simulink model "VDSE_2018a"  (R2018a)
settings: Solver=ode5  StartTime=0.0  StopTime=T_simulation  FixedStep=simulation_step_time  RelTol=1e-3
values from neighbouring files (symbols this model uses):
  A = 2    [vehicle_parameters_script.m]
  bump_height = 0    [vehicle_parameters_script.m]
  bump_length = 1    [vehicle_parameters_script.m]
  bump_time = 1    [vehicle_parameters_script.m]
  Bxf = 17.156    [BCD_Parameters.m]
  Bxr = 17.156    [BCD_Parameters.m]
  Byf = 12.71    [BCD_Parameters.m]
  Byr = 12.71    [BCD_Parameters.m]
  cd = 0.35    [vehicle_parameters_script.m]
  central_diff = 1    [vehicle_parameters_script.m]
  cF = 5000    [vehicle_parameters_script.m]
  clF = -0.15    [vehicle_parameters_script.m]
  clR = -0.20    (= -0.2)    [vehicle_parameters_script.m]
  cp_FA = 30    [vehicle_parameters_script.m]
  cp_RA = 13    [vehicle_parameters_script.m]
  cR = 5000    [vehicle_parameters_script.m]
  ctF = tireF.VERTICAL_DAMPING    [vehicle_parameters_script.m]
  ctR = tireR.VERTICAL_DAMPING    [vehicle_parameters_script.m]
  Cxf = 1.406    [BCD_Parameters.m]
  Cxr = 1.406    [BCD_Parameters.m]
  Cyf = 1.63    [BCD_Parameters.m]
  Cyr = 1.63    [BCD_Parameters.m]
  Dxf = 1.2    [BCD_Parameters.m]
  Dxr = 1.2    [BCD_Parameters.m]
  Dyf = 1.1    [BCD_Parameters.m]
  Dyr = 1.8    [BCD_Parameters.m]
  enableDriverControl = 0    [vehicle_parameters_script.m]
  enableLongDynamics = 1    [vehicle_parameters_script.m]
  enablePowertrain = 1    [vehicle_parameters_script.m]
  front_dr = 3.8    [vehicle_parameters_script.m]
  g = 9.806    [vehicle_parameters_script.m]
  Gear_numbers = [1 2 3 4 5 6]    [vehicle_parameters_script.m]
  GR = [2.9 1.8 1.3 1 0.85 0.75]    [vehicle_parameters_script.m]
  hcog = 0.5    [vehicle_parameters_script.m]
  hpc = 0.0    (= 0)    [vehicle_parameters_script.m]
  hrcF = 0.3    [vehicle_parameters_script.m]
  hrcg = (hrcF*lR+hrcR*lF)/(lF+lR)    (= 0.25108)    [vehicle_parameters_script.m]
  hrcR = 0.2    [vehicle_parameters_script.m]
  huFcog = 0.32    [vehicle_parameters_script.m]
  huRcog = 0.32    [vehicle_parameters_script.m]
  initial_gear = 1    [vehicle_parameters_script.m]
  JwF = 2.45    [vehicle_parameters_script.m]
  JwR = 2.45    [vehicle_parameters_script.m]
  Jx = 430    [vehicle_parameters_script.m]
  Jy = 1309    [vehicle_parameters_script.m]
  Jz = 1461    [vehicle_parameters_script.m]
  kF = 40000    [vehicle_parameters_script.m]
  kR = 35000    [vehicle_parameters_script.m]
  kRF = 0    [vehicle_parameters_script.m]
  kRR = 0    [vehicle_parameters_script.m]
  ktF = tireF.VERTICAL_STIFFNESS    [vehicle_parameters_script.m]
  ktR = tireR.VERTICAL_STIFFNESS    [vehicle_parameters_script.m]
  lF = 1.223    [vehicle_parameters_script.m]
  lR = l-lF    (= 1.277)    [vehicle_parameters_script.m]
  m = 1310    [vehicle_parameters_script.m]
  max_pressure = 1000    [vehicle_parameters_script.m]
  maxrpm = 4000    [vehicle_parameters_script.m]
  mF = 45    [vehicle_parameters_script.m]
  minrpm = 1500    [vehicle_parameters_script.m]
  mR = 50    [vehicle_parameters_script.m]
  output_samping_time = 0.001    [vehicle_parameters_script.m]
  phi0 = 0    [vehicle_parameters_script.m]
  phi_dot0 = 0    [vehicle_parameters_script.m]
  psi0 = 0    [vehicle_parameters_script.m]
  psi_dot0 = 0    [vehicle_parameters_script.m]
  rear_dr = 3.8    [vehicle_parameters_script.m]
  requested_speed = 100/3.6    (= 27.7777777778)    [vehicle_parameters_script.m]
  rF = tireF.UNLOADED_RADIUS    [vehicle_parameters_script.m]
  rho = 1.2    [vehicle_parameters_script.m]
  RPMME = Engine(:,1)    [vehicle_parameters_script.m]
  rR = tireR.UNLOADED_RADIUS    [vehicle_parameters_script.m]
  steer_ratio = 13.25    [vehicle_parameters_script.m]
  TFL = 0    [vehicle_parameters_script.m]
  TFR = 0    [vehicle_parameters_script.m]
  theta0 = 0    [vehicle_parameters_script.m]
  theta_dot0 = 0    [vehicle_parameters_script.m]
  TorqueME = []    [vehicle_parameters_script.m]
  TRL = 0    [vehicle_parameters_script.m]
  TRR = 0    [vehicle_parameters_script.m]
  Vx0 = 100/3.6    (= 27.7777777778)    [vehicle_parameters_script.m]
  Vy0 = 0    [vehicle_parameters_script.m]
  Vz0 = 0    [vehicle_parameters_script.m]
  wF = 1.578    [vehicle_parameters_script.m]
  wR = 1.544    [vehicle_parameters_script.m]
  x0 = 0    [vehicle_parameters_script.m]
  xcog_overall = (2*mR*xR+2*xF*mF+m*xs)/(m+2*mF+2*mR)    (= 1.23475333333)    [vehicle_parameters_script.m]
  y0 = 0    [vehicle_parameters_script.m]
  z0 = 0    [vehicle_parameters_script.m]
  zFL0 = 0    [vehicle_parameters_script.m]
  zFL_dot0 = 0    [vehicle_parameters_script.m]
  zFR0 = 0    [vehicle_parameters_script.m]
  zFR_dot0 = 0    [vehicle_parameters_script.m]
  zRL0 = 0    [vehicle_parameters_script.m]
  zRL_dot0 = 0    [vehicle_parameters_script.m]
  zRR0 = 0    [vehicle_parameters_script.m]
  zRR_dot0 = 0    [vehicle_parameters_script.m]
undefined symbols (not defined in the file or in its folder): exf, exr, eyf, eyr, FNOMINf, FNOMINr, PCX1f, PCX1r, PCY1f, PCY1r, PDX1f, PDX1r, PDX2f, PDX2r, PDY1f, PDY1r, PDY2f, PDY2r, PDY3f, PDY3r, PEX1f, PEX1r, PEX2f, PEX2r, PEX3f, PEX3r, PEX4f, PEX4r, PEY1f, PEY1r, PEY2f, PEY2r, PEY3f, PEY3r, PEY4f, PEY4r, PHX1f, PHX1r, PHX2f, PHX2r, PHY1f, PHY1r, PHY2f, PHY2r, PHY3f, PHY3r, PKX1f, PKX1r, PKX2f, PKX2r, PKX3f, PKX3r, PKY1f, PKY1r, PKY2f, PKY2r, PKY3f, PKY3r, PVX1f, PVX1r ... (+122)
libraries: simulink x7, mfeval_LIB x4
(part 4 of 6)

== system VDSE_2018a/14-DOF VEHICLE MODEL/WHEEL ASSEMBLY/WHEEL ASSEMBLY PACEIJKA/TIRE PARAMETERS ==
  Mux1 : Mux  Inputs=91
  Mux2 : Mux  Inputs=91
  TIRE PARAMETERS - FRONT AXLE : Subsystem
  TIRE PARAMETERS - REAR AXLE : Subsystem
  Tire Parameters Front Axle : Outport
  Tire Parameters Rear Axle : Outport  Port=2
  wires:
  TIRE PARAMETERS - FRONT AXLE/29(PCY1) -> Mux1/29
  TIRE PARAMETERS - FRONT AXLE/18(PKY3) -> Mux1/18
  TIRE PARAMETERS - FRONT AXLE/1(PHX1) -> Mux1/1
  TIRE PARAMETERS - FRONT AXLE/48(RVY4) -> Mux1/48
  TIRE PARAMETERS - FRONT AXLE/41(RBY1) -> Mux1/41
  TIRE PARAMETERS - FRONT AXLE/8(PEX3) -> Mux1/8
  TIRE PARAMETERS - FRONT AXLE/23(PHY1) -> Mux1/23
  TIRE PARAMETERS - FRONT AXLE/46(RVY2) -> Mux1/46
  TIRE PARAMETERS - FRONT AXLE/5(PCX1) -> Mux1/5
  TIRE PARAMETERS - FRONT AXLE/19(PVY1) -> Mux1/19
  TIRE PARAMETERS - FRONT AXLE/22(PVY4) -> Mux1/22
  TIRE PARAMETERS - FRONT AXLE/53(RHY1) -> Mux1/53
  TIRE PARAMETERS - FRONT AXLE/7(PEX2) -> Mux1/7
  TIRE PARAMETERS - FRONT AXLE/37(RCX1) -> Mux1/37
  TIRE PARAMETERS - FRONT AXLE/51(REY1) -> Mux1/51
  TIRE PARAMETERS - FRONT AXLE/28(PDY3) -> Mux1/28
  TIRE PARAMETERS - FRONT AXLE/36(RBX2) -> Mux1/36
  TIRE PARAMETERS - FRONT AXLE/34(ey) -> Mux1/34
  TIRE PARAMETERS - FRONT AXLE/10(PKX1) -> Mux1/10
  TIRE PARAMETERS - FRONT AXLE/30(PEY1) -> Mux1/30
  TIRE PARAMETERS - FRONT AXLE/17(PKY2) -> Mux1/17
  TIRE PARAMETERS - FRONT AXLE/2(PHX2) -> Mux1/2
  TIRE PARAMETERS - FRONT AXLE/33(PEY4) -> Mux1/33
  TIRE PARAMETERS - FRONT AXLE/39(REX2) -> Mux1/39
  TIRE PARAMETERS - FRONT AXLE/45(RVY1) -> Mux1/45
  TIRE PARAMETERS - FRONT AXLE/52(REY2) -> Mux1/52
  TIRE PARAMETERS - FRONT AXLE/21(PVY3) -> Mux1/21
  TIRE PARAMETERS - FRONT AXLE/3(PDX1) -> Mux1/3
  TIRE PARAMETERS - FRONT AXLE/6(PEX1) -> Mux1/6
  TIRE PARAMETERS - FRONT AXLE/4(PDX2) -> Mux1/4
  TIRE PARAMETERS - FRONT AXLE/49(RVY5) -> Mux1/49
  TIRE PARAMETERS - FRONT AXLE/44(RCY1) -> Mux1/44
  TIRE PARAMETERS - FRONT AXLE/25(PHY3) -> Mux1/25
  TIRE PARAMETERS - FRONT AXLE/24(PHY2) -> Mux1/24
  TIRE PARAMETERS - FRONT AXLE/54(RHY2) -> Mux1/54
  TIRE PARAMETERS - FRONT AXLE/43(RBY3) -> Mux1/43
  TIRE PARAMETERS - FRONT AXLE/13(ex) -> Mux1/13
  TIRE PARAMETERS - FRONT AXLE/31(PEY2) -> Mux1/31
  TIRE PARAMETERS - FRONT AXLE/14(PVX1) -> Mux1/14
  TIRE PARAMETERS - FRONT AXLE/35(RBX1) -> Mux1/35
  TIRE PARAMETERS - FRONT AXLE/15(PVX2) -> Mux1/15
  TIRE PARAMETERS - FRONT AXLE/27(PDY2) -> Mux1/27
  TIRE PARAMETERS - FRONT AXLE/20(PVY2) -> Mux1/20
  TIRE PARAMETERS - FRONT AXLE/11(PKX2) -> Mux1/11
  TIRE PARAMETERS - FRONT AXLE/50(RVY6) -> Mux1/50
  TIRE PARAMETERS - FRONT AXLE/32(PEY3) -> Mux1/32
  Mux1/1 -> Tire Parameters Front Axle/1
  TIRE PARAMETERS - FRONT AXLE/47(RVY3) -> Mux1/47
  TIRE PARAMETERS - FRONT AXLE/9(PEX4) -> Mux1/9
  TIRE PARAMETERS - FRONT AXLE/40(RHX1) -> Mux1/40
  TIRE PARAMETERS - FRONT AXLE/38(REX1) -> Mux1/38
  TIRE PARAMETERS - FRONT AXLE/42(RBY2) -> Mux1/42
  TIRE PARAMETERS - FRONT AXLE/26(PDY1) -> Mux1/26
  TIRE PARAMETERS - FRONT AXLE/12(PKX3) -> Mux1/12
  TIRE PARAMETERS - FRONT AXLE/16(PKY1) -> Mux1/16
  TIRE PARAMETERS - REAR AXLE/16(PKY1) -> Mux2/16
  TIRE PARAMETERS - REAR AXLE/12(PKX3) -> Mux2/12
  TIRE PARAMETERS - REAR AXLE/26(PDY1) -> Mux2/26
  TIRE PARAMETERS - REAR AXLE/42(RBY2) -> Mux2/42
  TIRE PARAMETERS - REAR AXLE/38(REX1) -> Mux2/38
  TIRE PARAMETERS - REAR AXLE/40(RHX1) -> Mux2/40
  TIRE PARAMETERS - REAR AXLE/9(PEX4) -> Mux2/9
  TIRE PARAMETERS - REAR AXLE/47(RVY3) -> Mux2/47
  Mux2/1 -> Tire Parameters Rear Axle/1
  TIRE PARAMETERS - REAR AXLE/32(PEY3) -> Mux2/32
  TIRE PARAMETERS - REAR AXLE/50(RVY6) -> Mux2/50
  TIRE PARAMETERS - REAR AXLE/11(PKX2) -> Mux2/11
  TIRE PARAMETERS - REAR AXLE/20(PVY2) -> Mux2/20
  TIRE PARAMETERS - REAR AXLE/27(PDY2) -> Mux2/27
  TIRE PARAMETERS - REAR AXLE/15(PVX2) -> Mux2/15
  TIRE PARAMETERS - REAR AXLE/35(RBX1) -> Mux2/35
  TIRE PARAMETERS - REAR AXLE/14(PVX1) -> Mux2/14
  TIRE PARAMETERS - REAR AXLE/31(PEY2) -> Mux2/31
  TIRE PARAMETERS - REAR AXLE/13(ex) -> Mux2/13
  TIRE PARAMETERS - REAR AXLE/43(RBY3) -> Mux2/43
  TIRE PARAMETERS - REAR AXLE/54(RHY2) -> Mux2/54
  TIRE PARAMETERS - REAR AXLE/24(PHY2) -> Mux2/24
  TIRE PARAMETERS - REAR AXLE/25(PHY3) -> Mux2/25
  TIRE PARAMETERS - REAR AXLE/44(RCY1) -> Mux2/44
  TIRE PARAMETERS - REAR AXLE/49(RVY5) -> Mux2/49
  TIRE PARAMETERS - REAR AXLE/4(PDX2) -> Mux2/4
  TIRE PARAMETERS - REAR AXLE/6(PEX1) -> Mux2/6
  TIRE PARAMETERS - REAR AXLE/3(PDX1) -> Mux2/3
  TIRE PARAMETERS - REAR AXLE/21(PVY3) -> Mux2/21
  TIRE PARAMETERS - REAR AXLE/52(REY2) -> Mux2/52
  TIRE PARAMETERS - REAR AXLE/45(RVY1) -> Mux2/45
  TIRE PARAMETERS - REAR AXLE/39(REX2) -> Mux2/39
  TIRE PARAMETERS - REAR AXLE/33(PEY4) -> Mux2/33
  TIRE PARAMETERS - REAR AXLE/2(PHX2) -> Mux2/2
  TIRE PARAMETERS - REAR AXLE/17(PKY2) -> Mux2/17
  TIRE PARAMETERS - REAR AXLE/30(PEY1) -> Mux2/30
  TIRE PARAMETERS - REAR AXLE/10(PKX1) -> Mux2/10
  TIRE PARAMETERS - REAR AXLE/34(ey) -> Mux2/34
  TIRE PARAMETERS - REAR AXLE/36(RBX2) -> Mux2/36
  TIRE PARAMETERS - REAR AXLE/28(PDY3) -> Mux2/28
  TIRE PARAMETERS - REAR AXLE/51(REY1) -> Mux2/51
  TIRE PARAMETERS - REAR AXLE/37(RCX1) -> Mux2/37
  TIRE PARAMETERS - REAR AXLE/7(PEX2) -> Mux2/7
  TIRE PARAMETERS - REAR AXLE/53(RHY1) -> Mux2/53
  TIRE PARAMETERS - REAR AXLE/22(PVY4) -> Mux2/22
  TIRE PARAMETERS - REAR AXLE/19(PVY1) -> Mux2/19
  TIRE PARAMETERS - REAR AXLE/5(PCX1) -> Mux2/5
  TIRE PARAMETERS - REAR AXLE/46(RVY2) -> Mux2/46
  TIRE PARAMETERS - REAR AXLE/23(PHY1) -> Mux2/23
  TIRE PARAMETERS - REAR AXLE/8(PEX3) -> Mux2/8
  TIRE PARAMETERS - REAR AXLE/41(RBY1) -> Mux2/41
  TIRE PARAMETERS - REAR AXLE/48(RVY4) -> Mux2/48
  TIRE PARAMETERS - REAR AXLE/1(PHX1) -> Mux2/1
  TIRE PARAMETERS - REAR AXLE/18(PKY3) -> Mux2/18
  TIRE PARAMETERS - REAR AXLE/29(PCY1) -> Mux2/29
  TIRE PARAMETERS - REAR AXLE/55(FNOMIN) -> Mux2/55
  TIRE PARAMETERS - FRONT AXLE/55(FNOMIN) -> Mux1/55
  TIRE PARAMETERS - FRONT AXLE/56(QHZ1) -> Mux1/56
  TIRE PARAMETERS - FRONT AXLE/57(QHZ2) -> Mux1/57
  TIRE PARAMETERS - FRONT AXLE/58(QHZ3) -> Mux1/58
  TIRE PARAMETERS - FRONT AXLE/59(QHZ4) -> Mux1/59
  TIRE PARAMETERS - FRONT AXLE/60(QBZ1) -> Mux1/60
  TIRE PARAMETERS - FRONT AXLE/61(QBZ2) -> Mux1/61
  TIRE PARAMETERS - FRONT AXLE/62(QBZ3) -> Mux1/62
  TIRE PARAMETERS - FRONT AXLE/63(QBZ4) -> Mux1/63
  TIRE PARAMETERS - FRONT AXLE/64(QBZ5) -> Mux1/64
  TIRE PARAMETERS - FRONT AXLE/65(QCZ1) -> Mux1/65
  TIRE PARAMETERS - FRONT AXLE/66(QDZ1) -> Mux1/66
  TIRE PARAMETERS - FRONT AXLE/67(QDZ2) -> Mux1/67
  TIRE PARAMETERS - FRONT AXLE/68(QDZ3) -> Mux1/68
  TIRE PARAMETERS - FRONT AXLE/69(QDZ4) -> Mux1/69
  TIRE PARAMETERS - FRONT AXLE/70(QEZ1) -> Mux1/70
  TIRE PARAMETERS - FRONT AXLE/71(QEZ2) -> Mux1/71
  TIRE PARAMETERS - FRONT AXLE/72(QEZ3) -> Mux1/72
  TIRE PARAMETERS - FRONT AXLE/73(QEZ4) -> Mux1/73
  TIRE PARAMETERS - FRONT AXLE/74(QEZ5) -> Mux1/74
  TIRE PARAMETERS - FRONT AXLE/75(QBZ9) -> Mux1/75
  TIRE PARAMETERS - FRONT AXLE/76(QBZ10) -> Mux1/76
  TIRE PARAMETERS - FRONT AXLE/77(QDZ6) -> Mux1/77
  TIRE PARAMETERS - FRONT AXLE/78(QDZ7) -> Mux1/78
  TIRE PARAMETERS - FRONT AXLE/79(QDZ8) -> Mux1/79
  TIRE PARAMETERS - FRONT AXLE/80(QDZ9) -> Mux1/80
  TIRE PARAMETERS - FRONT AXLE/81(R0) -> Mux1/81
  TIRE PARAMETERS - FRONT AXLE/82(zeta7) -> Mux1/82
  TIRE PARAMETERS - FRONT AXLE/83(SSZ1) -> Mux1/83
  TIRE PARAMETERS - FRONT AXLE/84(SSZ2) -> Mux1/84
  TIRE PARAMETERS - FRONT AXLE/85(SSZ3) -> Mux1/85
  TIRE PARAMETERS - FRONT AXLE/86(SSZ4) -> Mux1/86
  TIRE PARAMETERS - FRONT AXLE/87(QSY1) -> Mux1/87
  TIRE PARAMETERS - FRONT AXLE/88(QSY2) -> Mux1/88
  TIRE PARAMETERS - FRONT AXLE/89(QSY3) -> Mux1/89
  TIRE PARAMETERS - FRONT AXLE/90(QSY4) -> Mux1/90
  TIRE PARAMETERS - FRONT AXLE/91(VREF) -> Mux1/91
  TIRE PARAMETERS - REAR AXLE/56(QHZ1) -> Mux2/56
  TIRE PARAMETERS - REAR AXLE/57(QHZ2) -> Mux2/57
  TIRE PARAMETERS - REAR AXLE/58(QHZ3) -> Mux2/58
  TIRE PARAMETERS - REAR AXLE/59(QHZ4) -> Mux2/59
  TIRE PARAMETERS - REAR AXLE/60(QBZ1) -> Mux2/60
  TIRE PARAMETERS - REAR AXLE/61(QBZ2) -> Mux2/61
  TIRE PARAMETERS - REAR AXLE/62(QBZ3) -> Mux2/62
  TIRE PARAMETERS - REAR AXLE/63(QBZ4) -> Mux2/63
  TIRE PARAMETERS - REAR AXLE/64(QBZ5) -> Mux2/64
  TIRE PARAMETERS - REAR AXLE/65(QCZ1) -> Mux2/65
  TIRE PARAMETERS - REAR AXLE/66(QDZ1) -> Mux2/66
  TIRE PARAMETERS - REAR AXLE/67(QDZ2) -> Mux2/67
  TIRE PARAMETERS - REAR AXLE/68(QDZ3) -> Mux2/68
  TIRE PARAMETERS - REAR AXLE/69(QDZ4) -> Mux2/69
  TIRE PARAMETERS - REAR AXLE/70(QEZ1) -> Mux2/70
  TIRE PARAMETERS - REAR AXLE/71(QEZ2) -> Mux2/71
  TIRE PARAMETERS - REAR AXLE/72(QEZ3) -> Mux2/72
  TIRE PARAMETERS - REAR AXLE/73(QEZ4) -> Mux2/73
  TIRE PARAMETERS - REAR AXLE/74(QEZ5) -> Mux2/74
  TIRE PARAMETERS - REAR AXLE/75(QBZ9) -> Mux2/75
  TIRE PARAMETERS - REAR AXLE/76(QBZ10) -> Mux2/76
  TIRE PARAMETERS - REAR AXLE/77(QDZ6) -> Mux2/77
  TIRE PARAMETERS - REAR AXLE/78(QDZ7) -> Mux2/78
  TIRE PARAMETERS - REAR AXLE/79(QDZ8) -> Mux2/79
  TIRE PARAMETERS - REAR AXLE/80(QDZ9) -> Mux2/80
  TIRE PARAMETERS - REAR AXLE/81(R0) -> Mux2/81
  TIRE PARAMETERS - REAR AXLE/82(zeta7) -> Mux2/82
  TIRE PARAMETERS - REAR AXLE/83(SSZ1) -> Mux2/83
  TIRE PARAMETERS - REAR AXLE/84(SSZ2) -> Mux2/84
  TIRE PARAMETERS - REAR AXLE/85(SSZ3) -> Mux2/85
  TIRE PARAMETERS - REAR AXLE/86(SSZ4) -> Mux2/86
  TIRE PARAMETERS - REAR AXLE/87(QSY1) -> Mux2/87
  TIRE PARAMETERS - REAR AXLE/88(QSY2) -> Mux2/88
  TIRE PARAMETERS - REAR AXLE/89(QSY3) -> Mux2/89
  TIRE PARAMETERS - REAR AXLE/90(QSY4) -> Mux2/90
  TIRE PARAMETERS - REAR AXLE/91(VREF) -> Mux2/91

== system VDSE_2018a/14-DOF VEHICLE MODEL/SUSPENSION/FRONT SUSPENSION/SUSPENSION FL/FL ==
  z [m] : Inport
  Vz [m/s] : Inport  Port=2
  phi [rad] : Inport  Port=3
  phi_dot [rad/s] : Inport  Port=4
  theta [rad] : Inport  Port=5
  theta_dot [rad/s] : Inport  Port=6
  zFR [m] : Inport  Port=7
  yFL_road [m] : Inport  Port=8
  Constant : Constant  Value=zFL_dot0
  Constant1 : Constant  Value=zFL0
  Constant10 : Constant  Value=ctF
  Constant2 : Constant  Value=cF
  Constant3 : Constant  Value=wF
  Constant4 : Constant  Value=lF
  Constant5 : Constant  Value=kF
  Constant6 : Constant  Value=kRF
  Constant7 : Constant  Value=ktF
  Constant8 : Constant  Value=mF
  Constant9 : Constant  Value=g
  Derivative : Derivative
  Integrator : Integrator  InitialConditionSource=external
  Integrator1 : Integrator  InitialConditionSource=external
  MATLAB Function : MATLAB Function  TreatAsAtomicUnit=on
  zFL [m] : Outport
  zFL_dot [m/s] : Outport  Port=2
  wires:
  Constant9/1 -> MATLAB Function/9(g)
  Constant8/1 -> MATLAB Function/1(mF)
  Constant7/1 -> MATLAB Function/5(ktF)
  Constant6/1 -> MATLAB Function/4(kRF)
  Constant5/1 -> MATLAB Function/3(kF)
  Constant4/1 -> MATLAB Function/8(lF)
  Constant3/1 -> MATLAB Function/7(wF)
  Constant2/1 -> MATLAB Function/2(cF)
  zFR [m]/1 -> MATLAB Function/18(zFR)
  theta_dot [rad/s]/1 -> MATLAB Function/17(theta_dot)
  theta [rad]/1 -> MATLAB Function/16(theta)
  phi [rad]/1 -> MATLAB Function/14(phi)
  z [m]/1 -> MATLAB Function/12(z)
  yFL_road [m]/1 -> Derivative/1, MATLAB Function/10(yFL_road)
  Integrator/1 -> zFL [m]/1, MATLAB Function/19(zFL)  "zFL"
  Integrator1/1 -> zFL_dot [m/s]/1, MATLAB Function/20(zFL_dot), Integrator/1  "zFL_dot"
  MATLAB Function/1(zFL_dot_dot) -> Integrator1/1  "zFL_dot_dot"
  Vz [m/s]/1 -> MATLAB Function/13(Vz)
  phi_dot [rad/s]/1 -> MATLAB Function/15(phi_dot)
  Constant/1 -> Integrator1/2
  Constant1/1 -> Integrator/2
  Constant10/1 -> MATLAB Function/6(ctF)
  Derivative/1 -> MATLAB Function/11(yFL_road_dot)

== system VDSE_2018a/14-DOF VEHICLE MODEL/SUSPENSION/FRONT SUSPENSION/SUSPENSION FL/TIRE VERTICAL DEFLECTION ==
  zFL [m] : Inport
  zFL_dot [m/s] : Inport  Port=2
  yFL_road [m] : Inport  Port=3
  Add : Sum  Inputs=+-
  Add1 : Sum  Inputs=+-
  Add2 : Sum
  Derivative : Derivative
  Gain : Gain  Gain=-ktF
  Gain1 : Gain  Gain=-ctF
  yFL_road [m]1 : InportShadow  Port=3
  fFLz [N] : Outport
  wires:
  yFL_road [m]/1 -> Add/2
  zFL [m]/1 -> Add/1
  Add/1 -> Gain/1  "tire deflection FL"
  Gain/1 -> Add2/1
  yFL_road [m]1/1 -> Derivative/1
  Derivative/1 -> Add1/2
  zFL_dot [m/s]/1 -> Add1/1
  Add1/1 -> Gain1/1  "tire vertical velocity FL"
  Gain1/1 -> Add2/2
  Add2/1 -> fFLz [N]/1

== system VDSE_2018a/14-DOF VEHICLE MODEL/SUSPENSION/FRONT SUSPENSION/SUSPENSION FR/FR ==
  z [m] : Inport
  Vz [m/s] : Inport  Port=2
  phi [rad] : Inport  Port=3
  phi_dot [rad/s] : Inport  Port=4
  theta [rad] : Inport  Port=5
  theta_dot [rad/s] : Inport  Port=6
  zFL [m] : Inport  Port=7
  yFR_road [m] : Inport  Port=8
  Constant : Constant  Value=zFR_dot0
  Constant1 : Constant  Value=zFR0
  Constant10 : Constant  Value=ctF
  Constant2 : Constant  Value=cF
  Constant3 : Constant  Value=wF
  Constant4 : Constant  Value=lF
  Constant5 : Constant  Value=kF
  Constant6 : Constant  Value=kRF
  Constant7 : Constant  Value=ktF
  Constant8 : Constant  Value=mF
  Constant9 : Constant  Value=g
  Derivative : Derivative
  Integrator : Integrator  InitialConditionSource=external
  Integrator1 : Integrator  InitialConditionSource=external
  MATLAB Function : MATLAB Function  TreatAsAtomicUnit=on
  zFR [m] : Outport
  zFR_dot [m/s] : Outport  Port=2
  wires:
  Constant9/1 -> MATLAB Function/9(g)
  Constant8/1 -> MATLAB Function/1(mF)
  Constant7/1 -> MATLAB Function/8(ktF)
  Constant6/1 -> MATLAB Function/6(kRF)
  Constant5/1 -> MATLAB Function/5(kF)
  Constant4/1 -> MATLAB Function/4(lF)
  Constant3/1 -> MATLAB Function/3(wF)
  Constant2/1 -> MATLAB Function/2(cF)
  zFL [m]/1 -> MATLAB Function/18(zFL)
  theta_dot [rad/s]/1 -> MATLAB Function/17(theta_dot)
  theta [rad]/1 -> MATLAB Function/16(theta)
  phi_dot [rad/s]/1 -> MATLAB Function/15(phi_dot)
  phi [rad]/1 -> MATLAB Function/14(phi)
  Vz [m/s]/1 -> MATLAB Function/13(Vz)
  yFR_road [m]/1 -> Derivative/1, MATLAB Function/10(yFR_road)
  Integrator/1 -> zFR [m]/1, MATLAB Function/19(zFR)  "zFR"
  Integrator1/1 -> MATLAB Function/20(zFR_dot), zFR_dot [m/s]/1, Integrator/1  "zFR_dot"
  MATLAB Function/1(zFR_dot_dot) -> Integrator1/1  "zFR_dot_dot"
  z [m]/1 -> MATLAB Function/12(z)
  Constant/1 -> Integrator1/2
  Constant1/1 -> Integrator/2
  Constant10/1 -> MATLAB Function/7(ctF)
  Derivative/1 -> MATLAB Function/11(yFR_road_dot)

== system VDSE_2018a/14-DOF VEHICLE MODEL/SUSPENSION/FRONT SUSPENSION/SUSPENSION FR/TIRE VERTICAL DEFLECTION ==
  zFR [m] : Inport
  zFR_dot [m/s] : Inport  Port=2
  yFR_road [m] : Inport  Port=3
  Add : Sum  Inputs=+-
  Add1 : Sum
  Add2 : Sum  Inputs=+-
  Derivative : Derivative
  Gain : Gain  Gain=-ktF
  Gain1 : Gain  Gain=-ctF
  yFR_road [m]1 : InportShadow  Port=3
  fFRz [N] : Outport
  wires:
  yFR_road [m]/1 -> Add/2
  zFR [m]/1 -> Add/1
  Add/1 -> Gain/1  "tire deflection FR"
  Gain/1 -> Add1/1
  yFR_road [m]1/1 -> Derivative/1
  Derivative/1 -> Add2/2
  zFR_dot [m/s]/1 -> Add2/1
  Add2/1 -> Gain1/1  "tire vertical velocity FR"
  Gain1/1 -> Add1/2
  Add1/1 -> fFRz [N]/1

== system VDSE_2018a/14-DOF VEHICLE MODEL/SUSPENSION/REAR SUSPENSION/SUSPENSION RL/RL ==
  z [m] : Inport
  Vz [m/s] : Inport  Port=2
  phi [rad] : Inport  Port=3
  phi_dot [rad/s] : Inport  Port=4
  theta [rad] : Inport  Port=5
  theta_dot [rad/s] : Inport  Port=6
  zRR [m] : Inport  Port=7
  yRL_road [m] : Inport  Port=8
  Constant : Constant  Value=zRL_dot0
  Constant1 : Constant  Value=zRL0
  Constant10 : Constant  Value=ctR
  Constant2 : Constant  Value=cR
  Constant3 : Constant  Value=wR
  Constant4 : Constant  Value=lR
  Constant5 : Constant  Value=kR
  Constant6 : Constant  Value=kRR
  Constant7 : Constant  Value=ktR
  Constant8 : Constant  Value=mR
  Constant9 : Constant  Value=g
  Derivative : Derivative
  Integrator : Integrator  InitialConditionSource=external
  Integrator1 : Integrator  InitialConditionSource=external
  MATLAB Function : MATLAB Function  TreatAsAtomicUnit=on
  zRL [m] : Outport
  zRL_dot [m/s] : Outport  Port=2
  wires:
  zRR [m]/1 -> MATLAB Function/18(zRR)
  theta_dot [rad/s]/1 -> MATLAB Function/17(theta_dot)
  theta [rad]/1 -> MATLAB Function/16(theta)
  phi_dot [rad/s]/1 -> MATLAB Function/15(phi_dot)
  phi [rad]/1 -> MATLAB Function/14(phi)
  Vz [m/s]/1 -> MATLAB Function/13(Vz)
  z [m]/1 -> MATLAB Function/12(z)
  yRL_road [m]/1 -> MATLAB Function/10(yRL_road), Derivative/1
  Constant3/1 -> MATLAB Function/2(wR)
  Constant2/1 -> MATLAB Function/4(cR)
  Constant4/1 -> MATLAB Function/3(lR)
  Constant5/1 -> MATLAB Function/5(kR)
  Constant6/1 -> MATLAB Function/6(kRR)
  Constant7/1 -> MATLAB Function/8(ktR)
  Constant9/1 -> MATLAB Function/9(g)
  Constant8/1 -> MATLAB Function/1(mR)
  Integrator/1 -> MATLAB Function/19(zRL), zRL [m]/1  "zRL"
  Integrator1/1 -> Integrator/1, zRL_dot [m/s]/1, MATLAB Function/20(zRL_dot)  "zRL_dot"
  MATLAB Function/1(zRL_dot_dot) -> Integrator1/1  "zRL_dot_dot"
  Constant/1 -> Integrator1/2
  Constant1/1 -> Integrator/2
  Derivative/1 -> MATLAB Function/11(yRL_road_dot)
  Constant10/1 -> MATLAB Function/7(ctR)

== system VDSE_2018a/14-DOF VEHICLE MODEL/SUSPENSION/REAR SUSPENSION/SUSPENSION RL/TIRE VERTICAL DEFLECTION ==
  zRL [m] : Inport
  zRL_dot [m/s] : Inport  Port=2
  yRL_road [m] : Inport  Port=3
  Add : Sum  Inputs=+-
  Add1 : Sum  Inputs=+-
  Add2 : Sum
  Derivative : Derivative
  Gain : Gain  Gain=-ktR
  Gain1 : Gain  Gain=-ctR
  yRL_road [m]1 : InportShadow  Port=3
  fRLz [N] : Outport
  wires:
  yRL_road [m]/1 -> Add/2
  zRL [m]/1 -> Add/1
  Add/1 -> Gain/1  "tire deflection RL"
  Gain/1 -> Add2/1
  zRL_dot [m/s]/1 -> Add1/1
  Derivative/1 -> Add1/2
  yRL_road [m]1/1 -> Derivative/1
  Add1/1 -> Gain1/1  "tire vertical velocity RL"
  Gain1/1 -> Add2/2
  Add2/1 -> fRLz [N]/1

== system VDSE_2018a/14-DOF VEHICLE MODEL/SUSPENSION/REAR SUSPENSION/SUSPENSION RR/RR ==
  z [m] : Inport
  Vz [m/s] : Inport  Port=2
  phi [rad] : Inport  Port=3
  phi_dot [rad/s] : Inport  Port=4
  theta [rad] : Inport  Port=5
  theta_dot [rad/s] : Inport  Port=6
  zRL [m] : Inport  Port=7
  yRR_road [m] : Inport  Port=8
  Constant : Constant  Value=zRR_dot0
  Constant1 : Constant  Value=zRR0
  Constant10 : Constant  Value=ctR
  Constant2 : Constant  Value=cR
  Constant3 : Constant  Value=wR
  Constant4 : Constant  Value=lR
  Constant5 : Constant  Value=kR
  Constant6 : Constant  Value=kRR
  Constant7 : Constant  Value=ktR
  Constant8 : Constant  Value=mR
  Constant9 : Constant  Value=g
  Derivative : Derivative
  Integrator : Integrator  InitialConditionSource=external
  Integrator1 : Integrator  InitialConditionSource=external
  MATLAB Function : MATLAB Function  TreatAsAtomicUnit=on
  zRR [m] : Outport
  zRR_dot [m/s] : Outport  Port=2
  wires:
  zRL [m]/1 -> MATLAB Function/18(zRL)
  theta_dot [rad/s]/1 -> MATLAB Function/17(theta_dot)
  theta [rad]/1 -> MATLAB Function/16(theta)
  phi_dot [rad/s]/1 -> MATLAB Function/15(phi_dot)
  phi [rad]/1 -> MATLAB Function/14(phi)
  Vz [m/s]/1 -> MATLAB Function/13(Vz)
  z [m]/1 -> MATLAB Function/12(z)
  yRR_road [m]/1 -> Derivative/1, MATLAB Function/10(yRR_road)
  Constant9/1 -> MATLAB Function/9(g)
  Constant4/1 -> MATLAB Function/3(lR)
  Constant5/1 -> MATLAB Function/5(kR)
  Constant6/1 -> MATLAB Function/6(kRR)
  Constant7/1 -> MATLAB Function/8(ktR)
  Constant8/1 -> MATLAB Function/1(mR)
  Constant3/1 -> MATLAB Function/2(wR)
  Constant2/1 -> MATLAB Function/4(cR)
  MATLAB Function/1(zRR_dot_dot) -> Integrator1/1  "zRR_dot_dot"
  Integrator/1 -> zRR [m]/1, MATLAB Function/19(zRR)  "zRR"
  Integrator1/1 -> MATLAB Function/20(zRR_dot), Integrator/1, zRR_dot [m/s]/1  "zRR_dot"
  Constant1/1 -> Integrator/2
  Constant/1 -> Integrator1/2
  Derivative/1 -> MATLAB Function/11(yRR_road_dot)
  Constant10/1 -> MATLAB Function/7(ctR)

== system VDSE_2018a/14-DOF VEHICLE MODEL/SUSPENSION/REAR SUSPENSION/SUSPENSION RR/TIRE VERTICAL DEFLECTION ==
  zRR [m] : Inport
  zRR_dot [m/s] : Inport  Port=2
  yRR_road [m] : Inport  Port=3
  Add : Sum  Inputs=+-
  Add1 : Sum  Inputs=+-
  Add2 : Sum
  Derivative : Derivative
  Gain : Gain  Gain=-ktR
  Gain1 : Gain  Gain=-ctR
  yRR_road [m]1 : InportShadow  Port=3
  fRRz [N] : Outport
  wires:
  yRR_road [m]/1 -> Add/2
  zRR [m]/1 -> Add/1
  Add/1 -> Gain/1  "tire deflection RR"
  Gain/1 -> Add2/1
  zRR_dot [m/s]/1 -> Add1/1
  yRR_road [m]1/1 -> Derivative/1
  Derivative/1 -> Add1/2
  Add1/1 -> Gain1/1  "tire vertical velocity RR"
  Gain1/1 -> Add2/2
  Add2/1 -> fRRz [N]/1

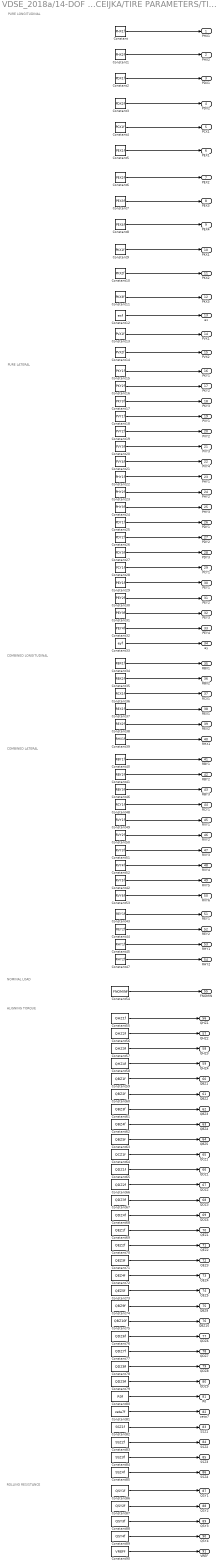
== system VDSE_2018a/14-DOF VEHICLE MODEL/WHEEL ASSEMBLY/WHEEL ASSEMBLY PACEIJKA/TIRE PARAMETERS/TIRE PARAMETERS - FRONT AXLE ==
  note: ALIGNING TORQUE
  note: ROLLING RESISTANCE
  note: PURE LONGITUDINAL
  note: PURE LATERAL
  note: COMBINED LATERAL
  note: COMBINED LONGITUDINAL
  note: NOMINAL LOAD
  Constant : Constant  Value=PHX1f
  Constant1 : Constant  Value=PHX2f
  Constant10 : Constant  Value=PKX2f
  Constant11 : Constant  Value=PKX3f
  Constant12 : Constant  Value=exf
  Constant13 : Constant  Value=PVX1f
  Constant14 : Constant  Value=PVX2f
  Constant15 : Constant  Value=PKY1f
  Constant16 : Constant  Value=PKY2f
  Constant17 : Constant  Value=PKY3f
  Constant18 : Constant  Value=PVY1f
  Constant19 : Constant  Value=PVY2f
  Constant2 : Constant  Value=PDX1f
  Constant20 : Constant  Value=PVY3f
  Constant21 : Constant  Value=PVY4f
  Constant22 : Constant  Value=PHY1f
  Constant23 : Constant  Value=PHY2f
  Constant24 : Constant  Value=PHY3f
  Constant25 : Constant  Value=PDY1f
  Constant26 : Constant  Value=PDY2f
  Constant27 : Constant  Value=PDY3f
  Constant28 : Constant  Value=PCY1f
  Constant29 : Constant  Value=PEY1f
  Constant3 : Constant  Value=PDX2f
  Constant30 : Constant  Value=PEY2f
  Constant31 : Constant  Value=PEY3f
  Constant32 : Constant  Value=PEY4f
  Constant33 : Constant  Value=eyf
  Constant34 : Constant  Value=RBX1f
  Constant35 : Constant  Value=RBX2f
  Constant36 : Constant  Value=RCX1f
  Constant37 : Constant  Value=REX1f
  Constant38 : Constant  Value=REX2f
  Constant39 : Constant  Value=RHX1f
  Constant4 : Constant  Value=PCX1f
  Constant40 : Constant  Value=RBY1f
  Constant41 : Constant  Value=RBY2f
  Constant42 : Constant  Value=RVY5f
  Constant43 : Constant  Value=REY1f
  Constant44 : Constant  Value=REY2f
  Constant45 : Constant  Value=RHY1f
  Constant46 : Constant  Value=RBY3f
  Constant47 : Constant  Value=RHY2f
  Constant48 : Constant  Value=RCY1f
  Constant49 : Constant  Value=RVY1f
  Constant5 : Constant  Value=PEX1f
  Constant50 : Constant  Value=RVY2f
  Constant51 : Constant  Value=RVY3f
  Constant52 : Constant  Value=RVY4f
  Constant53 : Constant  Value=RVY6f
  Constant54 : Constant  Value=FNOMINf
  Constant55 : Constant  Value=QHZ1f
  Constant56 : Constant  Value=QHZ2f
  Constant57 : Constant  Value=QHZ3f
  Constant58 : Constant  Value=QHZ4f
  Constant59 : Constant  Value=QBZ1f
  Constant6 : Constant  Value=PEX2f
  Constant60 : Constant  Value=QBZ2f
  Constant61 : Constant  Value=QBZ3f
  Constant62 : Constant  Value=QBZ4f
  Constant63 : Constant  Value=QBZ5f
  Constant64 : Constant  Value=QCZ1f
  Constant65 : Constant  Value=QDZ1f
  Constant66 : Constant  Value=QDZ2f
  Constant67 : Constant  Value=QDZ3f
  Constant68 : Constant  Value=QDZ4f
  Constant69 : Constant  Value=QEZ1f
  Constant7 : Constant  Value=PEX3f
  Constant70 : Constant  Value=QEZ2f
  Constant71 : Constant  Value=QEZ3f
  Constant72 : Constant  Value=QEZ4f
  Constant73 : Constant  Value=QEZ5f
  Constant74 : Constant  Value=QBZ9f
  Constant75 : Constant  Value=QBZ10f
  Constant76 : Constant  Value=QDZ6f
  Constant77 : Constant  Value=QDZ7f
  Constant78 : Constant  Value=QDZ8f
  Constant79 : Constant  Value=QDZ9f
  Constant8 : Constant  Value=PEX4f
  Constant80 : Constant  Value=R0f
  Constant81 : Constant  Value=zeta7f
  Constant82 : Constant  Value=SSZ1f
  Constant83 : Constant  Value=SSZ2f
  Constant84 : Constant  Value=SSZ3f
  Constant85 : Constant  Value=SSZ4f
  Constant86 : Constant  Value=QSY1f
  Constant87 : Constant  Value=QSY2f
  Constant88 : Constant  Value=QSY3f
  Constant89 : Constant  Value=QSY4f
  Constant9 : Constant  Value=PKX1f
  Constant90 : Constant  Value=VREFf
  PHX1 : Outport
  PHX2 : Outport  Port=2
  PDX1 : Outport  Port=3
  PDX2 : Outport  Port=4
  PCX1 : Outport  Port=5
  PEX1 : Outport  Port=6
  PEX2 : Outport  Port=7
  PEX3 : Outport  Port=8
  PEX4 : Outport  Port=9
  PKX1 : Outport  Port=10
  PKX2 : Outport  Port=11
  PKX3 : Outport  Port=12
  ex : Outport  Port=13
  PVX1 : Outport  Port=14
  PVX2 : Outport  Port=15
  PKY1 : Outport  Port=16
  PKY2 : Outport  Port=17
  PKY3 : Outport  Port=18
  PVY1 : Outport  Port=19
  PVY2 : Outport  Port=20
  PVY3 : Outport  Port=21
  PVY4 : Outport  Port=22
  PHY1 : Outport  Port=23
  PHY2 : Outport  Port=24
  PHY3 : Outport  Port=25
  PDY1 : Outport  Port=26
  PDY2 : Outport  Port=27
  PDY3 : Outport  Port=28
  PCY1 : Outport  Port=29
  PEY1 : Outport  Port=30
  PEY2 : Outport  Port=31
  PEY3 : Outport  Port=32
  PEY4 : Outport  Port=33
  ey : Outport  Port=34
  RBX1 : Outport  Port=35
  RBX2 : Outport  Port=36
  RCX1 : Outport  Port=37
  REX1 : Outport  Port=38
  REX2 : Outport  Port=39
  RHX1 : Outport  Port=40
  RBY1 : Outport  Port=41
  RBY2 : Outport  Port=42
  RBY3 : Outport  Port=43
  RCY1 : Outport  Port=44
  RVY1 : Outport  Port=45
  RVY2 : Outport  Port=46
  RVY3 : Outport  Port=47
  RVY4 : Outport  Port=48
  RVY5 : Outport  Port=49
  RVY6 : Outport  Port=50
  REY1 : Outport  Port=51
  REY2 : Outport  Port=52
  RHY1 : Outport  Port=53
  RHY2 : Outport  Port=54
  FNOMIN : Outport  Port=55
  QHZ1 : Outport  Port=56
  QHZ2 : Outport  Port=57
  QHZ3 : Outport  Port=58
  QHZ4 : Outport  Port=59
  QBZ1 : Outport  Port=60
  QBZ2 : Outport  Port=61
  QBZ3 : Outport  Port=62
  QBZ4 : Outport  Port=63
  QBZ5 : Outport  Port=64
  QCZ1 : Outport  Port=65
  QDZ1 : Outport  Port=66
  QDZ2 : Outport  Port=67
  QDZ3 : Outport  Port=68
  QDZ4 : Outport  Port=69
  QEZ1 : Outport  Port=70
  QEZ2 : Outport  Port=71
  QEZ3 : Outport  Port=72
  QEZ4 : Outport  Port=73
  QEZ5 : Outport  Port=74
  QBZ9 : Outport  Port=75
  QBZ10 : Outport  Port=76
  QDZ6 : Outport  Port=77
  QDZ7 : Outport  Port=78
  QDZ8 : Outport  Port=79
  QDZ9 : Outport  Port=80
  R0 : Outport  Port=81
  zeta7 : Outport  Port=82
  SSZ1 : Outport  Port=83
  SSZ2 : Outport  Port=84
  SSZ3 : Outport  Port=85
  SSZ4 : Outport  Port=86
  QSY1 : Outport  Port=87
  QSY2 : Outport  Port=88
  QSY3 : Outport  Port=89
  QSY4 : Outport  Port=90
  VREF : Outport  Port=91
  wires:
  Constant6/1 -> PEX2/1
  Constant7/1 -> PEX3/1
  Constant8/1 -> PEX4/1
  Constant11/1 -> PKX3/1
  Constant10/1 -> PKX2/1
  Constant9/1 -> PKX1/1
  Constant3/1 -> PDX2/1
  Constant4/1 -> PCX1/1
  Constant5/1 -> PEX1/1
  Constant2/1 -> PDX1/1
  Constant1/1 -> PHX2/1
  Constant/1 -> PHX1/1
  Constant12/1 -> ex/1
  Constant13/1 -> PVX1/1
  Constant14/1 -> PVX2/1
  Constant15/1 -> PKY1/1
  Constant16/1 -> PKY2/1
  Constant17/1 -> PKY3/1
  Constant18/1 -> PVY1/1
  Constant19/1 -> PVY2/1
  Constant20/1 -> PVY3/1
  Constant21/1 -> PVY4/1
  Constant22/1 -> PHY1/1
  Constant23/1 -> PHY2/1
  Constant24/1 -> PHY3/1
  Constant25/1 -> PDY1/1
  Constant26/1 -> PDY2/1
  Constant27/1 -> PDY3/1
  Constant28/1 -> PCY1/1
  Constant29/1 -> PEY1/1
  Constant30/1 -> PEY2/1
  Constant31/1 -> PEY3/1
  Constant32/1 -> PEY4/1
  Constant33/1 -> ey/1
  Constant34/1 -> RBX1/1
  Constant35/1 -> RBX2/1
  Constant36/1 -> RCX1/1
  Constant37/1 -> REX1/1
  Constant38/1 -> REX2/1
  Constant39/1 -> RHX1/1
  Constant45/1 -> RHY1/1
  Constant44/1 -> REY2/1
  Constant43/1 -> REY1/1
  Constant42/1 -> RVY5/1
  Constant41/1 -> RBY2/1
  Constant40/1 -> RBY1/1
  Constant46/1 -> RBY3/1
  Constant47/1 -> RHY2/1
  Constant48/1 -> RCY1/1
  Constant49/1 -> RVY1/1
  Constant50/1 -> RVY2/1
  Constant51/1 -> RVY3/1
  Constant52/1 -> RVY4/1
  Constant53/1 -> RVY6/1
  Constant54/1 -> FNOMIN/1
  Constant55/1 -> QHZ1/1
  Constant56/1 -> QHZ2/1
  Constant57/1 -> QHZ3/1
  Constant58/1 -> QHZ4/1
  Constant59/1 -> QBZ1/1
  Constant60/1 -> QBZ2/1
  Constant61/1 -> QBZ3/1
  Constant62/1 -> QBZ4/1
  Constant63/1 -> QBZ5/1
  Constant64/1 -> QCZ1/1
  Constant65/1 -> QDZ1/1
  Constant66/1 -> QDZ2/1
  Constant67/1 -> QDZ3/1
  Constant68/1 -> QDZ4/1
  Constant69/1 -> QEZ1/1
  Constant70/1 -> QEZ2/1
  Constant71/1 -> QEZ3/1
  Constant72/1 -> QEZ4/1
  Constant73/1 -> QEZ5/1
  Constant74/1 -> QBZ9/1
  Constant75/1 -> QBZ10/1
  Constant76/1 -> QDZ6/1
  Constant77/1 -> QDZ7/1
  Constant78/1 -> QDZ8/1
  Constant79/1 -> QDZ9/1
  Constant80/1 -> R0/1
  Constant81/1 -> zeta7/1
  Constant82/1 -> SSZ1/1
  Constant83/1 -> SSZ2/1
  Constant84/1 -> SSZ3/1
  Constant85/1 -> SSZ4/1
  Constant86/1 -> QSY1/1
  Constant87/1 -> QSY2/1
  Constant88/1 -> QSY3/1
  Constant89/1 -> QSY4/1
  Constant90/1 -> VREF/1

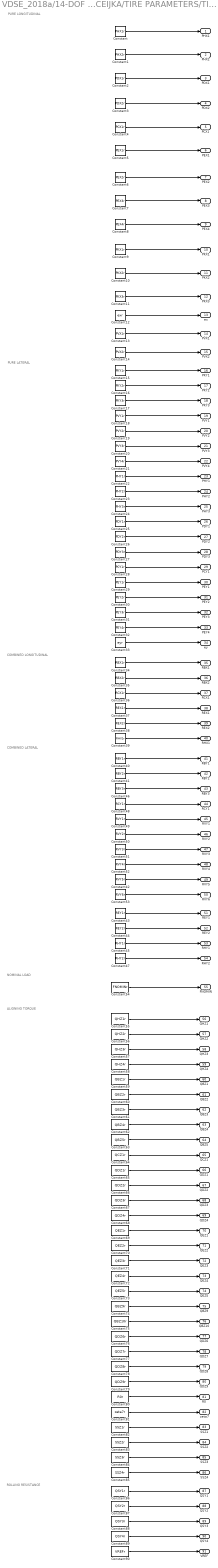
== system VDSE_2018a/14-DOF VEHICLE MODEL/WHEEL ASSEMBLY/WHEEL ASSEMBLY PACEIJKA/TIRE PARAMETERS/TIRE PARAMETERS - REAR AXLE ==
  note: NOMINAL LOAD
  note: COMBINED LONGITUDINAL
  note: COMBINED LATERAL
  note: PURE LATERAL
  note: PURE LONGITUDINAL
  note: ALIGNING TORQUE
  note: ROLLING RESISTANCE
  Constant : Constant  Value=PHX1r
  Constant1 : Constant  Value=PHX2r
  Constant10 : Constant  Value=PKX2r
  Constant11 : Constant  Value=PKX3r
  Constant12 : Constant  Value=exr
  Constant13 : Constant  Value=PVX1r
  Constant14 : Constant  Value=PVX2r
  Constant15 : Constant  Value=PKY1r
  Constant16 : Constant  Value=PKY2r
  Constant17 : Constant  Value=PKY3r
  Constant18 : Constant  Value=PVY1r
  Constant19 : Constant  Value=PVY2r
  Constant2 : Constant  Value=PDX1r
  Constant20 : Constant  Value=PVY3r
  Constant21 : Constant  Value=PVY4r
  Constant22 : Constant  Value=PHY1r
  Constant23 : Constant  Value=PHY2r
  Constant24 : Constant  Value=PHY3r
  Constant25 : Constant  Value=PDY1r
  Constant26 : Constant  Value=PDY2r
  Constant27 : Constant  Value=PDY3r
  Constant28 : Constant  Value=PCY1r
  Constant29 : Constant  Value=PEY1r
  Constant3 : Constant  Value=PDX2r
  Constant30 : Constant  Value=PEY2r
  Constant31 : Constant  Value=PEY3r
  Constant32 : Constant  Value=PEY4r
  Constant33 : Constant  Value=eyr
  Constant34 : Constant  Value=RBX1r
  Constant35 : Constant  Value=RBX2r
  Constant36 : Constant  Value=RCX1r
  Constant37 : Constant  Value=REX1r
  Constant38 : Constant  Value=REX2r
  Constant39 : Constant  Value=RHX1r
  Constant4 : Constant  Value=PCX1r
  Constant40 : Constant  Value=RBY1r
  Constant41 : Constant  Value=RBY2r
  Constant42 : Constant  Value=RVY5r
  Constant43 : Constant  Value=REY1r
  Constant44 : Constant  Value=REY2r
  Constant45 : Constant  Value=RHY1r
  Constant46 : Constant  Value=RBY3r
  Constant47 : Constant  Value=RHY2r
  Constant48 : Constant  Value=RCY1r
  Constant49 : Constant  Value=RVY1r
  Constant5 : Constant  Value=PEX1r
  Constant50 : Constant  Value=RVY2r
  Constant51 : Constant  Value=RVY3r
  Constant52 : Constant  Value=RVY4r
  Constant53 : Constant  Value=RVY6r
  Constant54 : Constant  Value=FNOMINr
  Constant55 : Constant  Value=QHZ1r
  Constant56 : Constant  Value=QHZ2r
  Constant57 : Constant  Value=QHZ3r
  Constant58 : Constant  Value=QHZ4r
  Constant59 : Constant  Value=QBZ1r
  Constant6 : Constant  Value=PEX2r
  Constant60 : Constant  Value=QBZ2r
  Constant61 : Constant  Value=QBZ3r
  Constant62 : Constant  Value=QBZ4r
  Constant63 : Constant  Value=QBZ5r
  Constant64 : Constant  Value=QCZ1r
  Constant65 : Constant  Value=QDZ1r
  Constant66 : Constant  Value=QDZ2r
  Constant67 : Constant  Value=QDZ3r
  Constant68 : Constant  Value=QDZ4r
  Constant69 : Constant  Value=QEZ1r
  Constant7 : Constant  Value=PEX3r
  Constant70 : Constant  Value=QEZ2r
  Constant71 : Constant  Value=QEZ3r
  Constant72 : Constant  Value=QEZ4r
  Constant73 : Constant  Value=QEZ5r
  Constant74 : Constant  Value=QBZ9r
  Constant75 : Constant  Value=QBZ10r
  Constant76 : Constant  Value=QDZ6r
  Constant77 : Constant  Value=QDZ7r
  Constant78 : Constant  Value=QDZ8r
  Constant79 : Constant  Value=QDZ9r
  Constant8 : Constant  Value=PEX4r
  Constant80 : Constant  Value=R0r
  Constant81 : Constant  Value=zeta7r
  Constant82 : Constant  Value=SSZ1r
  Constant83 : Constant  Value=SSZ2r
  Constant84 : Constant  Value=SSZ3r
  Constant85 : Constant  Value=SSZ4r
  Constant86 : Constant  Value=QSY1r
  Constant87 : Constant  Value=QSY2r
  Constant88 : Constant  Value=QSY3r
  Constant89 : Constant  Value=QSY4r
  Constant9 : Constant  Value=PKX1r
  Constant90 : Constant  Value=VREFr
  PHX1 : Outport
  PHX2 : Outport  Port=2
  PDX1 : Outport  Port=3
  PDX2 : Outport  Port=4
  PCX1 : Outport  Port=5
  PEX1 : Outport  Port=6
  PEX2 : Outport  Port=7
  PEX3 : Outport  Port=8
  PEX4 : Outport  Port=9
  PKX1 : Outport  Port=10
  PKX2 : Outport  Port=11
  PKX3 : Outport  Port=12
  ex : Outport  Port=13
  PVX1 : Outport  Port=14
  PVX2 : Outport  Port=15
  PKY1 : Outport  Port=16
  PKY2 : Outport  Port=17
  PKY3 : Outport  Port=18
  PVY1 : Outport  Port=19
  PVY2 : Outport  Port=20
  PVY3 : Outport  Port=21
  PVY4 : Outport  Port=22
  PHY1 : Outport  Port=23
  PHY2 : Outport  Port=24
  PHY3 : Outport  Port=25
  PDY1 : Outport  Port=26
  PDY2 : Outport  Port=27
  PDY3 : Outport  Port=28
  PCY1 : Outport  Port=29
  PEY1 : Outport  Port=30
  PEY2 : Outport  Port=31
  PEY3 : Outport  Port=32
  PEY4 : Outport  Port=33
  ey : Outport  Port=34
  RBX1 : Outport  Port=35
  RBX2 : Outport  Port=36
  RCX1 : Outport  Port=37
  REX1 : Outport  Port=38
  REX2 : Outport  Port=39
  RHX1 : Outport  Port=40
  RBY1 : Outport  Port=41
  RBY2 : Outport  Port=42
  RBY3 : Outport  Port=43
  RCY1 : Outport  Port=44
  RVY1 : Outport  Port=45
  RVY2 : Outport  Port=46
  RVY3 : Outport  Port=47
  RVY4 : Outport  Port=48
  RVY5 : Outport  Port=49
  RVY6 : Outport  Port=50
  REY1 : Outport  Port=51
  REY2 : Outport  Port=52
  RHY1 : Outport  Port=53
  RHY2 : Outport  Port=54
  FNOMIN : Outport  Port=55
  QHZ1 : Outport  Port=56
  QHZ2 : Outport  Port=57
  QHZ3 : Outport  Port=58
  QHZ4 : Outport  Port=59
  QBZ1 : Outport  Port=60
  QBZ2 : Outport  Port=61
  QBZ3 : Outport  Port=62
  QBZ4 : Outport  Port=63
  QBZ5 : Outport  Port=64
  QCZ1 : Outport  Port=65
  QDZ1 : Outport  Port=66
  QDZ2 : Outport  Port=67
  QDZ3 : Outport  Port=68
  QDZ4 : Outport  Port=69
  QEZ1 : Outport  Port=70
  QEZ2 : Outport  Port=71
  QEZ3 : Outport  Port=72
  QEZ4 : Outport  Port=73
  QEZ5 : Outport  Port=74
  QBZ9 : Outport  Port=75
  QBZ10 : Outport  Port=76
  QDZ6 : Outport  Port=77
  QDZ7 : Outport  Port=78
  QDZ8 : Outport  Port=79
  QDZ9 : Outport  Port=80
  R0 : Outport  Port=81
  zeta7 : Outport  Port=82
  SSZ1 : Outport  Port=83
  SSZ2 : Outport  Port=84
  SSZ3 : Outport  Port=85
  SSZ4 : Outport  Port=86
  QSY1 : Outport  Port=87
  QSY2 : Outport  Port=88
  QSY3 : Outport  Port=89
  QSY4 : Outport  Port=90
  VREF : Outport  Port=91
  wires:
  Constant53/1 -> RVY6/1
  Constant52/1 -> RVY4/1
  Constant51/1 -> RVY3/1
  Constant50/1 -> RVY2/1
  Constant49/1 -> RVY1/1
  Constant48/1 -> RCY1/1
  Constant47/1 -> RHY2/1
  Constant46/1 -> RBY3/1
  Constant40/1 -> RBY1/1
  Constant41/1 -> RBY2/1
  Constant42/1 -> RVY5/1
  Constant43/1 -> REY1/1
  Constant44/1 -> REY2/1
  Constant45/1 -> RHY1/1
  Constant39/1 -> RHX1/1
  Constant38/1 -> REX2/1
  Constant37/1 -> REX1/1
  Constant36/1 -> RCX1/1
  Constant35/1 -> RBX2/1
  Constant34/1 -> RBX1/1
  Constant33/1 -> ey/1
  Constant32/1 -> PEY4/1
  Constant31/1 -> PEY3/1
  Constant30/1 -> PEY2/1
  Constant29/1 -> PEY1/1
  Constant28/1 -> PCY1/1
  Constant27/1 -> PDY3/1
  Constant26/1 -> PDY2/1
  Constant25/1 -> PDY1/1
  Constant24/1 -> PHY3/1
  Constant23/1 -> PHY2/1
  Constant22/1 -> PHY1/1
  Constant21/1 -> PVY4/1
  Constant20/1 -> PVY3/1
  Constant19/1 -> PVY2/1
  Constant18/1 -> PVY1/1
  Constant17/1 -> PKY3/1
  Constant16/1 -> PKY2/1
  Constant15/1 -> PKY1/1
  Constant14/1 -> PVX2/1
  Constant13/1 -> PVX1/1
  Constant12/1 -> ex/1
  Constant/1 -> PHX1/1
  Constant1/1 -> PHX2/1
  Constant2/1 -> PDX1/1
  Constant5/1 -> PEX1/1
  Constant4/1 -> PCX1/1
  Constant3/1 -> PDX2/1
  Constant9/1 -> PKX1/1
  Constant10/1 -> PKX2/1
  Constant11/1 -> PKX3/1
  Constant8/1 -> PEX4/1
  Constant7/1 -> PEX3/1
  Constant6/1 -> PEX2/1
  Constant54/1 -> FNOMIN/1
  Constant64/1 -> QCZ1/1
  Constant69/1 -> QEZ1/1
  Constant80/1 -> R0/1
  Constant86/1 -> QSY1/1
  Constant77/1 -> QDZ7/1
  Constant58/1 -> QHZ4/1
  Constant81/1 -> zeta7/1
  Constant74/1 -> QBZ9/1
  Constant59/1 -> QBZ1/1
  Constant70/1 -> QEZ2/1
  Constant78/1 -> QDZ8/1
  Constant60/1 -> QBZ2/1
  Constant83/1 -> SSZ2/1
  Constant61/1 -> QBZ3/1
  Constant76/1 -> QDZ6/1
  Constant68/1 -> QDZ4/1
  Constant67/1 -> QDZ3/1
  Constant88/1 -> QSY3/1
  Constant84/1 -> SSZ3/1
  Constant75/1 -> QBZ10/1
  Constant90/1 -> VREF/1
  Constant85/1 -> SSZ4/1
  Constant65/1 -> QDZ1/1
  Constant72/1 -> QEZ4/1
  Constant87/1 -> QSY2/1
  Constant89/1 -> QSY4/1
  Constant79/1 -> QDZ9/1
  Constant56/1 -> QHZ2/1
  Constant57/1 -> QHZ3/1
  Constant82/1 -> SSZ1/1
  Constant62/1 -> QBZ4/1
  Constant71/1 -> QEZ3/1
  Constant63/1 -> QBZ5/1
  Constant73/1 -> QEZ5/1
  Constant55/1 -> QHZ1/1
  Constant66/1 -> QDZ2/1

== matlab function VDSE_2018a/14-DOF VEHICLE MODEL/SUSPENSION/Load Transfer/Tire lift from the ground check ==
  data: FLz_Overall input; FLz output; FRz_Overall input; RLz_Overall input; RRz_Overall input; ax input; ay input; FRz output; RLz output; RRz output; time input; trackwidth input; wheelbase input
function [FLz,FRz,RLz,RRz] = LiftFromGroundCheck(FLz_Overall,FRz_Overall,RLz_Overall,RRz_Overall,ax,ay,time, trackwidth, wheelbase)
                
if(time<1e-3)
    FLz=FLz_Overall;
    FRz=FRz_Overall;
    RLz=RLz_Overall;
    RRz=RRz_Overall;
    return
end
ax=abs(ax/wheelbase);
ay=abs(ay/trackwidth);
prop_lat=ay/(ax+ay);
prop_long=ax/(ax+ay);
FLz=FLz_Overall;
FRz=FRz_Overall;
RLz=RLz_Overall;
RRz=RRz_Overall;
fz_out = [FLz FRz RLz RRz];

while(min(fz_out)<0)
    [i,j] = find(fz_out <0);
    if(~isempty(find(j == 1)))
        if(fz_out(2) ==0)
            fz_out(4) = fz_out(4) + prop_lat*fz_out(1);
            fz_out(3) = fz_out(3) + prop_long*fz_out(1);
            fz_out(1) = 0;
        elseif (fz_out(3) ==0)
            fz_out(2) = fz_out(2) + prop_lat*fz_out(1);
            fz_out(4) = fz_out(4) + prop_long*fz_out(1);
            fz_out(1) = 0;
        else
        fz_out(2) = fz_out(2) + prop_lat*fz_out(1); %FRz=FRz_Overall+prop_lat*FLz_Overall;
        fz_out(3) = fz_out(3) + prop_long*fz_out(1); %RLz=RLz_Overall+prop_long*FLz_Overall;
        fz_out(1) = 0;
        end
    end
    
    if(~isempty(find(j == 2)))
        if(fz_out(1) ==0)
            fz_out(4) = fz_out(4) + prop_long*fz_out(2);
            fz_out(3) = fz_out(1) + prop_lat*fz_out(2);
            fz_out(2) = 0;
        elseif (fz_out(4) ==0)
            fz_out(1) = fz_out(1) + prop_lat*fz_out(2);
            fz_out(3) = fz_out(3) + prop_long*fz_out(2);
            fz_out(2) = 0;
        else
        fz_out(1) = fz_out(1) + prop_lat*fz_out(2); %FLz=FLz_Overall+prop_lat*FRz_Overall;
        fz_out(4) = fz_out(4) + prop_long*fz_out(2); %RRz=RRz_Overall+prop_long*FRz_Overall;
        fz_out(2) = 0;
        end
    end
    
    if(~isempty(find(j == 3)))
        if(fz_out(1) ==0)
            fz_out(4) = fz_out(4) + prop_lat*fz_out(3);
            fz_out(2) = fz_out(2) + prop_long*fz_out(3);
            fz_out(3) = 0;
        elseif (fz_out(4) ==0)
            fz_out(1) = fz_out(1) + prop_long*fz_out(3);
            fz_out(2) = fz_out(2) + prop_lat*fz_out(3);
            fz_out(3) = 0;
        else        
        fz_out(4) = fz_out(4) + prop_lat*fz_out(3);%RRz=RRz_Overall+prop_lat*RLz_Overall;
        fz_out(1) = fz_out(1) + prop_long*fz_out(3);%FLz=FLz_Overall+prop_long*RLz_Overall;
        fz_out(3) = 0;
        end
    end
    
    if(~isempty(find(j == 4)))
        if(fz_out(3) == 0)
            fz_out(2) = fz_out(2) +  prop_long*fz_out(4);
            fz_out(1) = fz_out(1) + prop_lat*fz_out(4);
            fz_out(4) = 0;
        elseif (fz_out(2) == 0)
            fz_out(3) = fz_out(3) + prop_lat*fz_out(2);
            fz_out(1) = fz_out(1) + prop_long*fz_out(4);
            fz_out(4) = 0;
        else        
        fz_out(3) =  fz_out(3) + prop_lat*fz_out(4);%RLz=RLz_Overall+prop_lat*RRz_Overall;
        fz_out(2) = fz_out(2) + prop_long*fz_out(4);%FRz=FRz_Overall+prop_long*RRz_Overall;
        fz_out(4) = 0;
        end
    end

end
FLz = fz_out(1);FRz = fz_out(2);RLz = fz_out(3);RRz = fz_out(4);
end

== matlab function VDSE_2018a/14-DOF VEHICLE MODEL/POWERTRAIN AND BRAKES/Engine and Gear Box/Subsystem1/MATLAB Function ==
  data: rpm input; gr_no output; gr_no_previous input; minrpm input; maxrpm input
function gr_no = Gear_change(rpm, gr_no_previous,minrpm, maxrpm)
gr_no = gr_no_previous;
if (rpm<=minrpm && gr_no > 1)
    gr_no = gr_no-1;
end
if (rpm >= maxrpm && gr_no<8)
    gr_no = gr_no+1;
end
end

== matlab function VDSE_2018a/14-DOF VEHICLE MODEL/SUSPENSION/FRONT SUSPENSION/SUSPENSION FL/FL/MATLAB Function ==
  data: mF input; cF input; kF input; kRF input; ktF input; ctF input; wF input; lF input; g input; yFL_road input; yFL_road_dot input; zFL_dot_dot output; z input; Vz input; phi input; phi_dot input; theta input; theta_dot input; zFR input; zFL input; zFL_dot input
function zFL_dot_dot = FL(mF,cF,kF,kRF,ktF,ctF,wF,lF,g,yFL_road,yFL_road_dot,z,Vz,phi,phi_dot,theta,theta_dot,zFR,zFL,zFL_dot)
% Parameters:
% mF = half front unsprung mass [kg]
% cF = front damping damping rate [Ns/m]
% kF = front spring stiffness [N/m]
% kRF = front antiroll bar stiffness [N/m]
% wF = front trackwidth [m]
% g = gravitational acceleration [m/s^2]
%
% Annotations:
% z = sprung mass vertical displacement [m]
% Vz = sprung mass vertical velocity [m/s]
% zij = unsprung vertical displacement [m]
% zij_dot = unsprung vertical velocity [m/s]
% zij_dot_dot = unsprung vertical acceleration [m/s^2]
% theta = pitch angle [rad]
% theta_dot = pitch angular velocity [rad/s]
% phi = roll angle [rad]
% phi_dot  = roll angular velocity [rad/s]
% y_front_road = front axle's road input displacement [m]
% y_front_road_dot = front axle's road input velocity [m/s]
%
% i: F, R = Front, Rear
% j: R, L = Right, Left

% Summation of forces:
sum = -cF*(Vz-zFL_dot+wF/2*phi_dot-lF*theta_dot) - kF*(z-zFL+wF/2*phi-lF*theta) - kRF/wF*(phi - (zFL-zFR)/wF) ...
    + ktF*(zFL-yFL_road)+ctF*(zFL_dot-yFL_road_dot)+mF*g;
% Calculation of FL unsprung mass vertical acceleration:
zFL_dot_dot = -sum/mF;
end

== matlab function VDSE_2018a/14-DOF VEHICLE MODEL/SUSPENSION/FRONT SUSPENSION/SUSPENSION FR/FR/MATLAB Function ==
  data: mF input; cF input; wF input; lF input; kF input; kRF input; ctF input; ktF input; g input; yFR_road input; yFR_road_dot input; zFR_dot_dot output; z input; Vz input; phi input; phi_dot input; theta input; theta_dot input; zFL input; zFR input; zFR_dot input
function zFR_dot_dot = FR(mF,cF,wF,lF,kF,kRF,ctF,ktF,g,yFR_road,yFR_road_dot, z, Vz, phi, phi_dot, theta, theta_dot, zFL,  zFR ,zFR_dot)
% Parameters:
% mF = half front unsprung mass [kg]
% cF = front damping damping rate [Ns/m]
% kF = front spring stiffness [N/m]
% kRF = front antiroll bar stiffness [N/m]
% wF = front trackwidth [m]
% g = gravitational acceleration [m/s^2]
%
% Annotations:
% z = sprung mass vertical displacement [m]
% Vz = sprung mass vertical velocity [m/s]
% zij = unsprung vertical displacement [m]
% zij_dot = unsprung vertical velocity [m/s]
% zij_dot_dot = unsprung vertical acceleration [m/s^2]
% theta = pitch angle [rad]
% theta_dot = pitch angular velocity [rad/s]
% phi = roll angle [rad]
% phi_dot  = roll angular velocity [rad/s]
% y_front_road = front axle's road input displacement [m]
% y_front_road_dot = front axle's road input velocity [m/s]
%
% i: F, R = Front, Rear
% j: R, L = Right, Left

% Summation of forces:
sum = -cF*(Vz-zFR_dot-wF/2*phi_dot-lF*theta_dot)-kF*(z-zFR-wF/2*phi-lF*theta)+kRF/wF*(phi-(zFL-zFR)/wF) ...
    +ktF*(zFR-yFR_road)+ctF*(zFR_dot-yFR_road_dot) + mF*g;

% Calculation of FR unsprung mass vertical acceleration:
zFR_dot_dot = -sum/mF;

end
